simulink model "airgk"  (Simulink 8.7)
settings: Solver=ode45  StartTime=0  StopTime=250  RelTol=1e-3
undefined symbols (not defined in the file or in its folder): GM1, x0, xfix
undefined symbols (not defined in the file): AM, GM2
libraries: airlib x1
(part 2 of 2)

== system airgk/Subsystem/eqm/xdotcorr ==
  xdot uncorrected : Inport
  yhlp : Inport  Port=2
  yatm : Inport  Port=3
  0 : Subsystem
      mask Display: disp('XDOTCORR (General)\nM.O. Rauw, October 1997')
  Demux : Demux  Outputs=12
  Mux1 : Mux  Inputs=12
  Mux2 : Mux  Inputs=[11 1 5]
  beta dot correction : Fcn  Expr=u[12] / (1 - (u[3]*u[13]*b*S*CYbdot)/(4*m))
  xdot corrected : Outport
  wires:
  beta dot correction/1 -> Mux1/3
  yatm/1 -> Mux2/3
  Demux/1 -> Mux1/1
  Demux/2 -> Mux1/2
  Demux/4 -> Mux1/4
  Demux/5 -> Mux1/5
  Demux/6 -> Mux1/6
  Demux/7 -> Mux1/7
  Demux/8 -> Mux1/8
  Demux/9 -> Mux1/9
  Demux/10 -> Mux1/10
  Demux/11 -> Mux1/11
  Demux/12 -> Mux1/12
  Demux/3 -> Mux2/2
  xdot uncorrected/1 -> Demux/1
  Mux1/1 -> xdot corrected/1
  Mux2/1 -> beta dot correction/1
  yhlp/1 -> Mux2/1

== system airgk/Subsystem/fms/0 ==

== system airgk/Subsystem/fw/0 ==

== system airgk/Subsystem/gr/0 ==

== system airgk/Subsystem/hlp/0 ==

== system airgk/Subsystem/out/0 ==

== system airgk/Subsystem/out/accel ==
  Ftot : Inport
  Fgrav : Inport  Port=2
  0 : Subsystem
      mask Display: disp('ACCEL\nM.O. Rauw, October 1997')
  Ax : Fcn  Expr=(u[1]-u[4])/(m*9.80665)
  Ay : Fcn  Expr=(u[2]-u[5])/(m*9.80665)
  Az : Fcn  Expr=(u[3]-u[6])/(m*9.80665)
  Mux : Mux  Inputs=6
  Mux1 : Mux  Inputs=[3 3]
  axk : Fcn  Expr=u[1]/(m*9.80665)
  ayk : Fcn  Expr=u[2]/(m*9.80665)
  azk : Fcn  Expr=u[3]/(m*9.80665)
  yacc : Outport
  wires:
  Ftot/1 -> Mux1/1
  Fgrav/1 -> Mux1/2
  Mux/1 -> yacc/1
  azk/1 -> Mux/6
  Az/1 -> Mux/3
  Ay/1 -> Mux/2
  Ax/1 -> Mux/1
  Mux1/1 -> Az/1, Ax/1, Ay/1, axk/1, azk/1, ayk/1
  axk/1 -> Mux/4
  ayk/1 -> Mux/5

== system airgk/Subsystem/out/fp ==
  x : Inport
  xdot : Inport  Port=2
  0 : Subsystem
      mask Display: disp('FLPATH\nM.O. Rauw, October 1997')
  Mux : Mux  Inputs=[12 12]
  Mux1 : Mux
  Phi : Fcn  Expr=u[9]*cos(u[8]-alpha0)
  chi : Fcn  Expr=u[3]+u[7]
  fpa : Fcn  Expr=u[13]/9.80665
  gamma : Fcn  Expr=asin(u[24]/u[1])
  yfp : Outport
  wires:
  gamma/1 -> Mux1/1
  Mux/1 -> chi/1, Phi/1, fpa/1, gamma/1
  fpa/1 -> Mux1/2
  chi/1 -> Mux1/3
  Phi/1 -> Mux1/4
  Mux1/1 -> yfp/1
  x/1 -> Mux/1
  xdot/1 -> Mux/2

== system airgk/Subsystem/out/uvwdot ==
  note: `
  note: cos(alpha)
  note: sin(alpha)
  note: cos(beta)
  note: sin(beta)
  note: V
  x : Inport
  xdot : Inport  Port=2
  yhlp : Inport  Port=3
  0 : Subsystem
      mask Display: disp('UVWDOT\nM.O. Rauw, October 1997')
  DeMux : Demux  Outputs=[1 1 1 1 7]
  Demux : Demux  Outputs=[1 11]
  Mux : Mux  Inputs=[1 1 1 1 1 12]
  Mux1 : Mux  Inputs=3
  Terminator : Terminator
  Terminator1 : Terminator
  u dot : Fcn  Expr=u[6]*u[1]*u[3] - u[5]*(u[7]*u[2]*u[3] + u[8]*u[1]*u[4])
  v dot : Fcn  Expr=u[6]*u[4] + u[5]*u[3]*u[8]
  wdot : Fcn  Expr=u[6]*u[2]*u[3] + u[5]*(u[7]*u[1]*u[3] - u[8]*u[2]*u[4])
  yuvw =  [udot; vdot; wdot] : Outport
  wires:
  Demux/2 -> Terminator1/1
  DeMux/5 -> Terminator/1
  wdot/1 -> Mux1/3
  v dot/1 -> Mux1/2
  u dot/1 -> Mux1/1
  xdot/1 -> Mux/6
  Mux/1 -> v dot/1, wdot/1, u dot/1
  DeMux/1 -> Mux/1
  DeMux/2 -> Mux/2
  x/1 -> Demux/1
  Mux1/1 -> yuvw =  [udot; vdot; wdot]/1
  yhlp/1 -> DeMux/1
  DeMux/3 -> Mux/3
  DeMux/4 -> Mux/4
  Demux/1 -> Mux/5

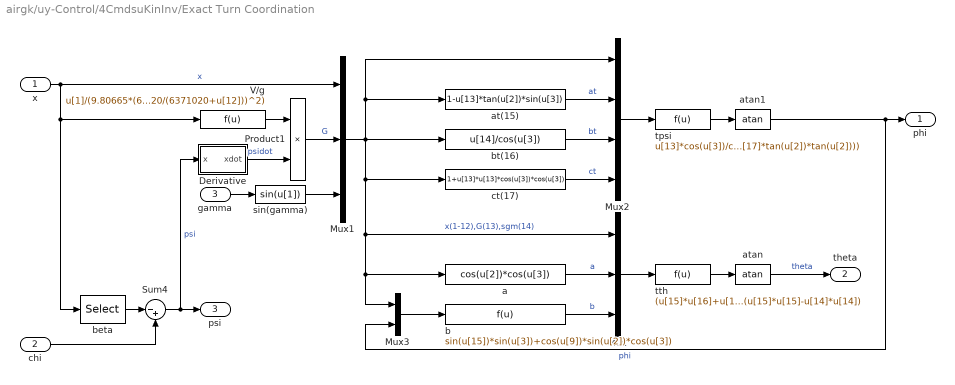
== system airgk/uy-Control/4CmdsuKinInv/Exact Turn Coordination ==
  x : Inport
  chi : Inport  Port=2
  gamma : Inport  Port=3
  Derivative : Subsystem  mask(Time Derivative){T=T, x0=Psi0}
      mask prompts: T "Sampling Time"; x0 "Initial Condition"
      mask help:
      | First order approximation of the time derivative of the input signal,
      |   the original one is buggy.
  Mux : Mux  Inputs=[14 1 1]
  Mux1 : Mux  Inputs=[12 1 1]
  Mux2 : Mux  Inputs=[14 1 1 1]
  Mux3 : Mux  Inputs=[14 1]
  Product1 : Product  Inputs=**  SaturateOnIntegerOverflow=on  RndMeth=Zero  InputSameDT=on  OutDataTypeStr=Inherit: Same as first input
  Sum4 : Sum  Inputs=|-+  SaturateOnIntegerOverflow=on  InputSameDT=on  OutDataTypeStr=Inherit: Same as first input
  V/g : Fcn  Expr=u[1]/(9.80665*(6371020/(6371020+u[12]))^2)
  a : Fcn  Expr=cos(u[2])*cos(u[3])
  at(15) : Fcn  Expr=1-u[13]*tan(u[2])*sin(u[3])
  atan : Trigonometry  Operator=atan
  atan1 : Trigonometry  Operator=atan
  b : Fcn  Expr=sin(u[15])*sin(u[3])+cos(u[9])*sin(u[2])*cos(u[3])
  beta : Selector  InputPortWidth=12  IndexOptions=Index vector (dialog)  Indices=3  OutputSizes=1
  bt(16) : Fcn  Expr=u[14]/cos(u[3])
  ct(17) : Fcn  Expr=1+u[13]*u[13]*cos(u[3])*cos(u[3])
  sin(gamma) : Fcn
  tpsi : Fcn  Expr=u[13]*cos(u[3])/cos(u[2])*(u[15]-u[16]*u[16]+u[16]*tan(u[2])*sqrt(abs(u[17]*(1-u[16]*u[16])+u[13]*u[13]*sin(u[3])*sin(u[3]))))/(u[15]*u[15]-u[16]*u[16]*(1+u[17]*tan(u[2])*tan(u[2])))
  tth : Fcn  Expr=(u[15]*u[16]+u[14]*sqrt(abs(u[15]*u[15]-u[14]*u[14]+u[16]*u[16])))/(u[15]*u[15]-u[14]*u[14])
  phi : Outport
  theta : Outport  Port=2
  psi : Outport  Port=3
  wires:
  Sum4/1 -> Derivative/1(x), psi/1  "psi"
  beta/1 -> Sum4/1
  chi/1 -> Sum4/2
  Derivative/1(xdot) -> Product1/2  "psidot"
  V/g/1 -> Product1/1
  gamma/1 -> sin(gamma)/1
  sin(gamma)/1 -> Mux1/3
  Product1/1 -> Mux1/2  "G"
  Mux1/1 -> bt(16)/1, at(15)/1, Mux2/1, ct(17)/1, Mux/1, a/1, Mux3/1  "x(1-12),G(13),sgm(14)"
  Mux2/1 -> tpsi/1
  tth/1 -> atan/1
  Mux/1 -> tth/1
  Mux3/1 -> b/1
  a/1 -> Mux/2  "a"
  b/1 -> Mux/3  "b"
  atan1/1 -> Mux3/2, phi/1  "phi"
  tpsi/1 -> atan1/1
  at(15)/1 -> Mux2/2  "at"
  bt(16)/1 -> Mux2/3  "bt"
  ct(17)/1 -> Mux2/4  "ct"
  atan/1 -> theta/1  "theta"
  x/1 -> beta/1, V/g/1, Mux1/1  "x"

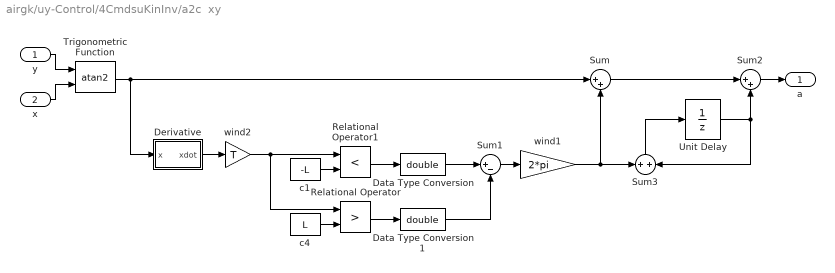
== system airgk/uy-Control/4CmdsuKinInv/a2c  xy ==
  y : Inport
  x : Inport  Port=2
  Data Type Conversion : DataTypeConversion  OutDataTypeStr=double  SaturateOnIntegerOverflow=on  RndMeth=Zero
  Data Type Conversion1 : DataTypeConversion  OutDataTypeStr=double  SaturateOnIntegerOverflow=on  RndMeth=Zero
  Derivative : Subsystem  mask(Time Derivative){T=T}
      mask prompts: T "Sampling Time"
      mask help:
      | First order approximation of the time derivative of the input signal,
      |   the original one is buggy.
  Relational Operator : RelationalOperator  Operator=>  InputSameDT=on
  Relational Operator1 : RelationalOperator  Operator=<  InputSameDT=on
  Sum : Sum  Inputs=|++  SaturateOnIntegerOverflow=on  InputSameDT=on  OutDataTypeStr=Inherit: Same as first input
  Sum1 : Sum  Inputs=|+-  SaturateOnIntegerOverflow=on  InputSameDT=on  OutDataTypeStr=Inherit: Same as first input
  Sum2 : Sum  Inputs=|++  SaturateOnIntegerOverflow=on  InputSameDT=on  OutDataTypeStr=Inherit: Same as first input
  Sum3 : Sum  SaturateOnIntegerOverflow=on  InputSameDT=on  OutDataTypeStr=Inherit: Same as first input
  Trigonometric Function : Trigonometry  Operator=atan2
  Unit Delay : UnitDelay  SampleTime=T
  c1 : Constant  Value=-L
  c4 : Constant  Value=L
  wind1 : Gain  Gain=2*pi  SaturateOnIntegerOverflow=on  OutDataTypeStr=Inherit: Same as input  ParamDataTypeStr=Inherit: Same as input
  wind2 : Gain  Gain=T  SaturateOnIntegerOverflow=on  OutDataTypeStr=Inherit: Same as input  ParamDataTypeStr=Inherit: Same as input
  a : Outport
  wires:
  Trigonometric Function/1 -> Sum/1, Derivative/1(x)
  Derivative/1(xdot) -> wind2/1
  wind2/1 -> Relational Operator/1, Relational Operator1/1
  c4/1 -> Relational Operator/2
  c1/1 -> Relational Operator1/2
  Relational Operator1/1 -> Data Type Conversion/1
  Relational Operator/1 -> Data Type Conversion1/1
  Data Type Conversion/1 -> Sum1/1
  Data Type Conversion1/1 -> Sum1/2
  Sum1/1 -> wind1/1
  wind1/1 -> Sum/2, Sum3/1
  Sum/1 -> Sum2/1
  Unit Delay/1 -> Sum2/2, Sum3/2
  Sum3/1 -> Unit Delay/1
  y/1 -> Trigonometric Function/1
  Sum2/1 -> a/1
  x/1 -> Trigonometric Function/2

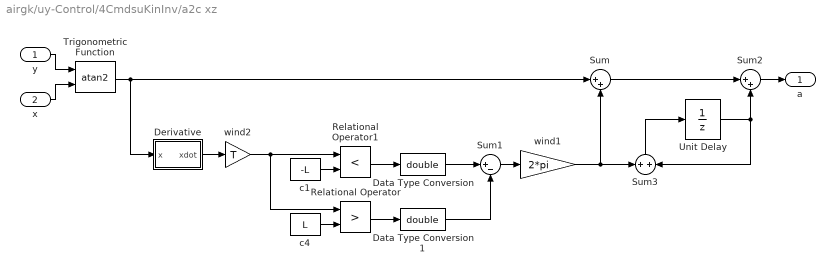
== system airgk/uy-Control/4CmdsuKinInv/a2c xz ==
  y : Inport
  x : Inport  Port=2
  Data Type Conversion : DataTypeConversion  OutDataTypeStr=double  SaturateOnIntegerOverflow=on  RndMeth=Zero
  Data Type Conversion1 : DataTypeConversion  OutDataTypeStr=double  SaturateOnIntegerOverflow=on  RndMeth=Zero
  Derivative : Subsystem  mask(Time Derivative){T=T}
      mask prompts: T "Sampling Time"
      mask help:
      | First order approximation of the time derivative of the input signal,
      |   the original one is buggy.
  Relational Operator : RelationalOperator  Operator=>  InputSameDT=on
  Relational Operator1 : RelationalOperator  Operator=<  InputSameDT=on
  Sum : Sum  Inputs=|++  SaturateOnIntegerOverflow=on  InputSameDT=on  OutDataTypeStr=Inherit: Same as first input
  Sum1 : Sum  Inputs=|+-  SaturateOnIntegerOverflow=on  InputSameDT=on  OutDataTypeStr=Inherit: Same as first input
  Sum2 : Sum  Inputs=|++  SaturateOnIntegerOverflow=on  InputSameDT=on  OutDataTypeStr=Inherit: Same as first input
  Sum3 : Sum  SaturateOnIntegerOverflow=on  InputSameDT=on  OutDataTypeStr=Inherit: Same as first input
  Trigonometric Function : Trigonometry  Operator=atan2
  Unit Delay : UnitDelay  SampleTime=T
  c1 : Constant  Value=-L
  c4 : Constant  Value=L
  wind1 : Gain  Gain=2*pi  SaturateOnIntegerOverflow=on  OutDataTypeStr=Inherit: Same as input  ParamDataTypeStr=Inherit: Same as input
  wind2 : Gain  Gain=T  SaturateOnIntegerOverflow=on  OutDataTypeStr=Inherit: Same as input  ParamDataTypeStr=Inherit: Same as input
  a : Outport
  wires:
  x/1 -> Trigonometric Function/2
  Sum2/1 -> a/1
  y/1 -> Trigonometric Function/1
  Sum3/1 -> Unit Delay/1
  Unit Delay/1 -> Sum3/2, Sum2/2
  Sum/1 -> Sum2/1
  wind1/1 -> Sum3/1, Sum/2
  Sum1/1 -> wind1/1
  Data Type Conversion1/1 -> Sum1/2
  Data Type Conversion/1 -> Sum1/1
  Relational Operator/1 -> Data Type Conversion1/1
  Relational Operator1/1 -> Data Type Conversion/1
  c1/1 -> Relational Operator1/2
  c4/1 -> Relational Operator/2
  wind2/1 -> Relational Operator1/1, Relational Operator/1
  Derivative/1(xdot) -> wind2/1
  Trigonometric Function/1 -> Derivative/1(x), Sum/1

== system airgk/uy-Control/Vcmd Generator/IIR1 ==
  In : Inport
  Discrete State-Space : DiscreteStateSpace  A=A  B=B  C=C  D=D  X0=x0  SampleTime=T
  Out : Outport
  wires:
  In/1 -> Discrete State-Space/1
  Discrete State-Space/1 -> Out/1

== system airgk/uy-Control/Vcmd Generator/IIR2 ==
  In : Inport
  Discrete State-Space : DiscreteStateSpace  A=A  B=B  C=C  D=D  X0=x0  SampleTime=T
  Out : Outport
  wires:
  In/1 -> Discrete State-Space/1
  Discrete State-Space/1 -> Out/1

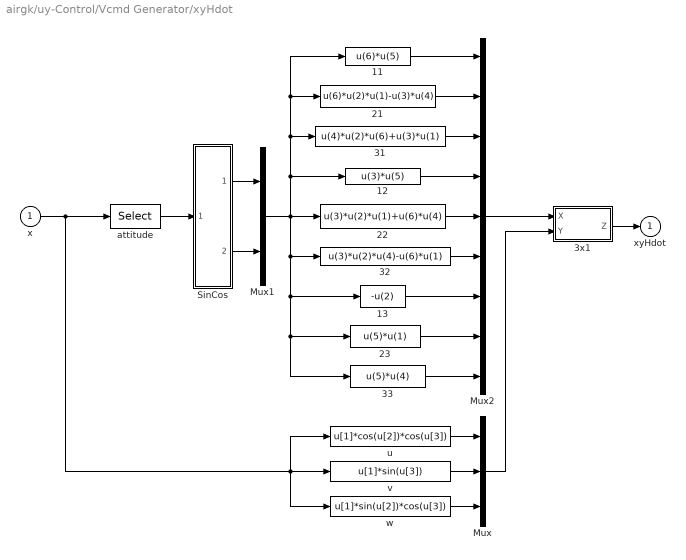
== system airgk/uy-Control/Vcmd Generator/xyHdot ==
  x : Inport
  11 : Fcn  Expr=u(6)*u(5)
  12 : Fcn  Expr=u(3)*u(5)
  13 : Fcn  Expr=-u(2)
  21 : Fcn  Expr=u(6)*u(2)*u(1)-u(3)*u(4)
  22 : Fcn  Expr=u(3)*u(2)*u(1)+u(6)*u(4)
  23 : Fcn  Expr=u(5)*u(1)
  31 : Fcn  Expr=u(4)*u(2)*u(6)+u(3)*u(1)
  32 : Fcn  Expr=u(3)*u(2)*u(4)-u(6)*u(1)
  33 : Fcn  Expr=u(5)*u(4)
  3x1 : Subsystem  mask(3x3 Matrix Multiplication){}
      mask help:
      | Input 1   : elements of matrix X (3 by 3)
      |   Input 2   : elements of matrix Y (3 by 3)
      |   Output   : elements of matrix X*Y (3 by 3)
      mask Help:
      | <p>
      | Elements of input and output matrices are taken columnwise.
      | </p>
      mask Display: disp('Z=X*Y')
  Mux : Mux  Inputs=3
  Mux1 : Mux  Inputs=2
  Mux2 : Mux  Inputs=9
  SinCos : Subsystem  mask(SinCos){}
      mask help: Compute the sine and cosine of input, u. u is in radians.
      mask Help: web(asbhelp);
      mask Display:
      | port_label('output',1,'sin(u)','texmode','on');
      | port_label('output',2,'cos(u)','texmode','on');
  attitude : Selector  InputPortWidth=12  IndexOptions=Index vector (dialog)  Indices=[9 8 7]  OutputSizes=1
  u : Fcn  Expr=u[1]*cos(u[2])*cos(u[3])
  v : Fcn  Expr=u[1]*sin(u[3])
  w : Fcn  Expr=u[1]*sin(u[2])*cos(u[3])
  xyHdot : Outport
  wires:
  x/1 -> attitude/1, v/1, w/1, u/1
  33/1 -> Mux2/9
  23/1 -> Mux2/8
  13/1 -> Mux2/7
  32/1 -> Mux2/6
  22/1 -> Mux2/5
  12/1 -> Mux2/4
  31/1 -> Mux2/3
  21/1 -> Mux2/2
  11/1 -> Mux2/1
  SinCos/1(sin(theta)) -> Mux1/1
  SinCos/2(cos(theta)) -> Mux1/2
  Mux1/1 -> 22/1, 11/1, 21/1, 31/1, 12/1, 32/1, 13/1, 23/1, 33/1
  attitude/1 -> SinCos/1(theta)
  w/1 -> Mux/3
  u/1 -> Mux/1
  v/1 -> Mux/2
  Mux/1 -> 3x1/2(Y)
  Mux2/1 -> 3x1/1(X)
  3x1/1(Z) -> xyHdot/1

== system airgk/uy-Control/uDynInv/ u term ==
  x : Inport
  udd : Inport  Port=2
  Mux1 : Mux  Inputs=[12 3 1]
  Term 1 with T=0 : Fcn  Expr=m*u[12+4]+m*(9.80665*(6371020/(6371020+u[12]))^2)*sin(u[8])+m*(u[5]*u[12+3]-u[6]*u[12+2])
  uvw : Subsystem  mask(uvw){}
      mask help:
      | Calculation of body-axes velocities
      | u, v, and w
      mask Help: eval('fdchelp uvw')
      mask Display: disp('Body-axes\nvelocities')
  mix : Outport
  wires:
  x/1 -> Mux1/1, uvw/1(x)
  Mux1/1 -> Term 1 with T=0/1
  Term 1 with T=0/1 -> mix/1
  uvw/1(ybvel) -> Mux1/2
  udd/1 -> Mux1/3

== system airgk/uy-Control/uDynInv/AM_CF ==
  In1 : Inport
  Matrix Gain : StateSpace  A=[]  B=[]  C=[]  D=M  X0=0
  Out1 : Outport
  wires:
  In1/1 -> Matrix Gain/1
  Matrix Gain/1 -> Out1/1

== system airgk/uy-Control/uDynInv/AM_SF ==
  In1 : Inport
  Matrix Gain : StateSpace  A=[]  B=[]  C=[]  D=M  X0=0
  Out1 : Outport
  wires:
  In1/1 -> Matrix Gain/1
  Matrix Gain/1 -> Out1/1

== system airgk/uy-Control/uDynInv/AM_SM ==
  In1 : Inport
  Matrix Gain : StateSpace  A=[]  B=[]  C=[]  D=M  X0=0
  Out1 : Outport
  wires:
  Matrix Gain/1 -> Out1/1
  In1/1 -> Matrix Gain/1

== system airgk/uy-Control/uDynInv/Inertia Products ==
  w : Inport
  wd : Inport  Port=2
  3x1mult : Subsystem  mask(3x1 Matrix Multiplication){}
      mask help:
      | Input 1   : elements of matrix X (3 by 3)
      |   Input 2   : elements of matrix Y (3 by 1)
      |   Output   : elements of matrix X*Y (3 by 1)
      mask Help:
      | <p>
      | Elements of input and output matrices are taken columnwise.
      | </p>
      mask Display: disp('Z=X*Y')
  3x1mult1 : Subsystem  mask(3x1 Matrix Multiplication){}
      mask help:
      | Input 1   : elements of matrix X (3 by 3)
      |   Input 2   : elements of matrix Y (3 by 1)
      |   Output   : elements of matrix X*Y (3 by 1)
      mask Help:
      | <p>
      | Elements of input and output matrices are taken columnwise.
      | </p>
      mask Display: disp('Z=X*Y')
  3x1mult2 : Subsystem  mask(3x1 Matrix Multiplication){}
      mask help:
      | Input 1   : elements of matrix X (3 by 3)
      |   Input 2   : elements of matrix Y (3 by 1)
      |   Output   : elements of matrix X*Y (3 by 1)
      mask Help:
      | <p>
      | Elements of input and output matrices are taken columnwise.
      | </p>
      mask Display: disp('Z=X*Y')
  Inertia Matrix : Constant  Value=[GM1(4) -GM1(7) -GM1(8) -GM1(7) GM1(5) -GM1(9) -GM1(8) -GM1(9) GM1(6)]
  Sum : Sum  Inputs=|++  SaturateOnIntegerOverflow=on  InputSameDT=on  OutDataTypeStr=Inherit: Same as first input
  w2W : Subsystem
      mask Display: disp('S')
  W*J*w+J*wt : Outport
  wires:
  w2W/1(Out1) -> 3x1mult2/1(X)
  3x1mult1/1(Z) -> 3x1mult2/2(Y)
  w/1 -> 3x1mult1/2(Y), w2W/1(In1)
  3x1mult/1(Z) -> Sum/1
  3x1mult2/1(Z) -> Sum/2
  Sum/1 -> W*J*w+J*wt/1
  wd/1 -> 3x1mult/2(Y)
  Inertia Matrix/1 -> 3x1mult/1(X), 3x1mult1/1(X)

== system airgk/uy-Control/uDynInv/Inv Rot ==
  w : Inport
  ftp : Inport  Port=2
  add : Inport  Port=3
  M : Subsystem  mask(Simulink Matrix Library Block){}
      mask help:
      | Roll, Pitch and Yaw derivatives to Omega :
      |   Input 1 : Roll, Pitch and Yaw angles (phi,theta,psi)
      |   Input 2 : Roll, Pitch and Yaw derivatives
      |   Output : Omega (p,q,r)
      mask Help:
      | <p>
      | Roll, Pitch and Yaw angles express the orientation
      | of the Body frame with respect to the Earth frame.
      | </p>
      | <p>
      | To use this block you should have the smxl library in your path.
      | </p>
  Sum1 : Sum  Inputs=+++  SaturateOnIntegerOverflow=on  InputSameDT=on  OutDataTypeStr=Inherit: Same as first input
  dM/df : Subsystem
  dM/dt : Subsystem
  pqr2ftpdot : Subsystem  mask(Simulink Matrix Library Block){}
      mask help:
      | Omega to Roll, Pitch and Yaw derivatives :
      |   Input 1 : Roll, Pitch and Yaw angles (phi,theta,psi)
      |   Input 2 : Omega (p,q,r)
      |   Output : Roll, Pitch and Yaw derivatives
      mask Help:
      | <p>
      | Roll, Pitch and Yaw angles express the orientation
      | of the Body frame with respect to the Earth frame.
      | </p>
      | <p>
      | To use this block you should have the smxl library in your path.
      | </p>
  wd : Outport
  wires:
  add/1 -> M/2(ftpdot)
  ftp/1 -> pqr2ftpdot/1(ftp), M/1(ftp), dM/df/1(ftp), dM/dt/1(ftp)
  w/1 -> pqr2ftpdot/2(pqr)
  pqr2ftpdot/1(ftpdot) -> dM/dt/2(ftpd), dM/df/2(ftpd)
  M/1(pqr) -> Sum1/3
  dM/dt/1(Tt) -> Sum1/1
  dM/df/1(Tf) -> Sum1/2
  Sum1/1 -> wd/1

== system airgk/uy-Control/uDynInv/ad1 ==
  x : Inport
  yatm : Inport  Port=2
  0 : Subsystem
      settings: OpenFcn=fdchelp airdata1
      mask Display: disp('AIRDATA1\nM.O. Rauw, October 1997')
  M : Fcn  Expr=u[2]/u[1]
  Mux : Mux  Inputs=[1 12]
  Mux1 : Mux  Inputs=[12 5]
  Mux2 : Mux  Inputs=3
  a : Fcn  Expr=sqrt(401.8743*u[3])
  qdyn : Fcn  Expr=0.5*u[13]*u[1]^2
  yad1 : Outport
  wires:
  yatm/1 -> Mux1/2, a/1
  x/1 -> Mux1/1, Mux/2
  Mux/1 -> M/1
  Mux1/1 -> qdyn/1
  M/1 -> Mux2/2
  a/1 -> Mux2/1, Mux/1
  qdyn/1 -> Mux2/3
  Mux2/1 -> yad1/1

== system airgk/uy-Control/uDynInv/atm ==
  x : Inport
  0 : Subsystem
      settings: OpenFcn=fdchelp atmosph
      mask Display: disp('ATMOSPH\nM.O. Rauw, October 1997')
  Mux : Mux  Inputs=2
  Mux1 : Mux  Inputs=[2 1]
  Mux2 : Mux  Inputs=5
  T : Fcn  Expr=288.15 - 0.0065*u[12]
  g : Fcn  Expr=9.80665*(6371020/(6371020+u[12]))^2
  mu : Fcn  Expr=(1.458*10^(-6)*u[2]^1.5)/(u[2]+110.4)
  ps : Fcn  Expr=101325*(u[2]/288.15)^(u[1]/1.86584)
  rho : Fcn  Expr=u[3]/(287.053*u[2])
  yatm : Outport
  wires:
  mu/1 -> Mux2/4
  Mux2/1 -> yatm/1
  Mux1/1 -> rho/1
  rho/1 -> Mux2/1
  g/1 -> Mux2/5, Mux/1
  T/1 -> Mux2/3, Mux/2
  ps/1 -> Mux2/2, Mux1/2
  Mux/1 -> ps/1, mu/1, Mux1/1
  x/1 -> g/1, T/1

== system airgk/uy-Control/uDynInv/dl ==
  x : Inport
  0 : Subsystem
      settings: OpenFcn=fdchelp dimless
      mask Display: disp('DIMLESS\nM.O. Rauw, October 1997')
  Mux : Mux  Inputs=3
  pb/2V : Fcn  Expr=0.5 * u[4] * b / u[1]
  qc/2V : Fcn  Expr=0.5* u[5] * cbar / u[1]
  rb/2V : Fcn  Expr=0.5 * u[6] * b / u[1]
  ydl : Outport
  wires:
  pb/2V/1 -> Mux/1
  qc/2V/1 -> Mux/2
  rb/2V/1 -> Mux/3
  Mux/1 -> ydl/1
  x/1 -> qc/2V/1, rb/2V/1, pb/2V/1

== system airgk/uy-Control/uDynInv/inv AM_CM ==
  In1 : Inport
  Matrix Gain : StateSpace  A=[]  B=[]  C=[]  D=M  X0=0
  Out1 : Outport
  wires:
  In1/1 -> Matrix Gain/1
  Matrix Gain/1 -> Out1/1

== system airgk/Subsystem/ad/ad1/0 ==

== system airgk/Subsystem/ad/atm/0 ==

== system airgk/Subsystem/ae/aero/0 ==

== system airgk/Subsystem/ae/aero/AM  ==
  In1 : Inport
  Matrix Gain : StateSpace  A=[]  B=[]  C=[]  D=M  X0=0
  Out1 : Outport
  wires:
  In1/1 -> Matrix Gain/1
  Matrix Gain/1 -> Out1/1

== system airgk/Subsystem/ae/aero/Stability 2 Body Axis ==
  alpha : Inport
  FsMb : Inport  Port=2
  Demux2 : Demux  Outputs=6
  Mux1 : Mux  Inputs=6
  Product{2..5} (4 alike) : Product  SaturateOnIntegerOverflow=on  RndMeth=Zero  InputSameDT=on  OutDataTypeStr=Inherit: Same as first input
  Sum3 : Sum  Inputs=-+  SaturateOnIntegerOverflow=on  InputSameDT=on  OutDataTypeStr=Inherit: Same as first input
  Sum4 : Sum  Inputs=--  SaturateOnIntegerOverflow=on  InputSameDT=on  OutDataTypeStr=Inherit: Same as first input
  cos alpha : Fcn  Expr=cos(u[1])
  sin alpha : Fcn
  FbMb : Outport
  wires:
  Demux2/6 -> Mux1/6
  Demux2/5 -> Mux1/5
  Demux2/2 -> Mux1/2
  Demux2/4 -> Mux1/4
  cos alpha/1 -> Product2/1, Product5/1
  Demux2/1 -> Product2/2, Product4/2
  Product2/1 -> Sum3/1
  Product3/1 -> Sum3/2
  Sum3/1 -> Mux1/1
  sin alpha/1 -> Product3/1, Product4/1
  Demux2/3 -> Product3/2, Product5/2
  Product4/1 -> Sum4/1
  Product5/1 -> Sum4/2
  Sum4/1 -> Mux1/3
  alpha/1 -> sin alpha/1, cos alpha/1
  Mux1/1 -> FbMb/1
  FsMb/1 -> Demux2/1

== system airgk/Subsystem/ae/dl/0 ==

== system airgk/Subsystem/ae/fmdims/0 ==

== system airgk/Subsystem/eqm/ODE/0 ==

== system airgk/Subsystem/eqm/ODE/Eulerdot ==
  note: ueul=[x;Ftot;Mtot;yhlp]
  note: yeul=[psi dot; theta dot; phi dot]
  ueul : Inport
  0 : Subsystem
      mask Display: disp('EULERDOT\nM.O. Rauw, October 1997')
  Mux1 : Mux  Inputs=[29 1]
  Mux2 : Mux  Inputs=3
  phi dot : Fcn  Expr=u[4] + u[30]*u[26]
  psi dot : Fcn  Expr=(u[5]*u[28] + u[6]*u[29])/u[27]
  theta dot : Fcn  Expr=u[5]*u[29] - u[6]*u[28]
  yeul : Outport
  wires:
  ueul/1 -> theta dot/1, Mux1/1, psi dot/1
  psi dot/1 -> Mux2/1, Mux1/2
  theta dot/1 -> Mux2/2
  Mux2/1 -> yeul/1
  phi dot/1 -> Mux2/3
  Mux1/1 -> phi dot/1

== system airgk/Subsystem/eqm/ODE/Vabdot ==
  note: yVab=[V dot;alpha dot;beta dot]
  note: uVab=[x;Ftot;Mtot;yhlp]
  uVab : Inport
  0 : Subsystem
      mask Display: disp('VABDOT\nM.O. Rauw, October 1997')
  Mux2 : Mux  Inputs=3
  V dot : Fcn  Expr=(u[13]*u[19]*u[21]+u[14]*u[22]+u[15]*u[20]*u[21])/m
  alpha dot : Fcn  Expr=(-u[13]*u[20]+u[15]*u[19])/(m*u[1]*u[21]) - u[23]*(u[4]*u[19]+u[6]*u[20]) + u[5]
  beta dot : Fcn  Expr=(-u[13]*u[19]*u[22]+u[14]*u[21]-u[15]*u[20]*u[22])/(m*u[1]) + u[4]*u[20] - u[6]*u[19]
  yVab : Outport
  wires:
  beta dot/1 -> Mux2/3
  V dot/1 -> Mux2/1
  alpha dot/1 -> Mux2/2
  uVab/1 -> alpha dot/1, beta dot/1, V dot/1
  Mux2/1 -> yVab/1

== system airgk/Subsystem/eqm/ODE/pqrdot ==
  note: ytmp = [L; M; N; p^2; pq; pr; q^2; qr; r^2]
  note: upqr=[x;Ftot;Mtot;yhlp]
  note: ypqr=[p dot;q dot;r dot]
  note: ytmp
  note: Here: ypqr = GM2*ytmp
  note: [L M N]'
  note: [p q r]'
  upqr : Inport
  0 : Subsystem
      mask Display: disp('PQRDOT\nM.O. Rauw, October 1997')
  Demux : Demux  Outputs=[3 3 9 3 11]
  Fcn : Fcn  Expr=u[1]^2
  Fcn1 : Fcn  Expr=u[1]*u[2]
  Fcn2 : Fcn  Expr=u[1]*u[3]
  Fcn3 : Fcn  Expr=u[2]^2
  Fcn4 : Fcn  Expr=u[2]*u[3]
  Fcn5 : Fcn  Expr=u[3]^2
  "GM2 " : Subsystem  mask(State Space){M=GM2}
      mask prompts: M "Matrix"
      mask Display: disp('Matrix\nGain')
  Mux : Mux  Inputs=[3 1 1 1 1 1 1]
  Terminator1 : Terminator
  Terminator2 : Terminator
  Terminator3 : Terminator
  ypqr : Outport
  wires:
  Mux/1 -> "GM2 "/1(In1)
  "GM2 "/1(Out1) -> ypqr/1
  Fcn5/1 -> Mux/7
  Fcn4/1 -> Mux/6
  Fcn3/1 -> Mux/5
  Fcn2/1 -> Mux/4
  Fcn1/1 -> Mux/3
  Fcn/1 -> Mux/2
  Demux/4 -> Mux/1
  Demux/2 -> Fcn3/1, Fcn5/1, Fcn4/1, Fcn2/1, Fcn/1, Fcn1/1
  Demux/3 -> Terminator1/1
  Demux/5 -> Terminator2/1
  Demux/1 -> Terminator3/1
  upqr/1 -> Demux/1

== system airgk/Subsystem/eqm/ODE/xyHdot ==
  note: uxyH=[x;Ftot;Mtot;yhlp]
  note: yxyH=[xe dot; ye dot; H dot]
  ybvel* : Inport
  uxYH : Inport  Port=2
  0 : Subsystem
      mask Display: disp('XYHDOT\nM.O. Rauw, October 1997')
  H dot : Fcn  Expr=u[30]*u[26] - (u[31]*u[28]+u[32]*u[29])*u[27]
  Mux2 : Mux  Inputs=[29 3]
  Mux3 : Mux  Inputs=2
  Mux4 : Mux  Inputs=[29 2]
  Mux5 : Mux  Inputs=3
  tmp1 : Fcn  Expr=u[30]*u[27] + (u[31]*u[28]+u[32]*u[29])*u[26]
  tmp2 : Fcn  Expr=u[31]*u[29] - u[32]*u[28]
  xe dot : Fcn  Expr=u[30]*u[25] - u[31]*u[24]
  ye dot : Fcn  Expr=u[30]*u[24] + u[31]*u[25]
  yxyH : Outport
  wires:
  uxYH/1 -> Mux2/1, Mux4/1
  ybvel*/1 -> Mux2/2
  Mux3/1 -> Mux4/2
  Mux2/1 -> tmp1/1, tmp2/1, H dot/1
  Mux4/1 -> xe dot/1, ye dot/1
  Mux5/1 -> yxyH/1
  ye dot/1 -> Mux5/2
  tmp2/1 -> Mux3/2
  xe dot/1 -> Mux5/1
  H dot/1 -> Mux5/3
  tmp1/1 -> Mux3/1

== system airgk/Subsystem/eqm/uvw/0 ==

== system airgk/Subsystem/eqm/xdotcorr/0 ==

== system airgk/Subsystem/out/accel/0 ==

== system airgk/Subsystem/out/fp/0 ==

== system airgk/Subsystem/out/uvwdot/0 ==

== system airgk/uy-Control/4CmdsuKinInv/Exact Turn Coordination/Derivative ==
  x : Inport
  Product2 : Product  Inputs=/*  SaturateOnIntegerOverflow=on  RndMeth=Zero  InputSameDT=on  OutDataTypeStr=Inherit: Same as first input
  Sum4 : Sum  Inputs=|+-  SaturateOnIntegerOverflow=on  InputSameDT=on  OutDataTypeStr=Inherit: Same as first input
  Unit Delay1 : UnitDelay  InitialCondition=x0  SampleTime=T
  Zero-Order Hold1 : ZeroOrderHold  SampleTime=T
  m : Constant  Value=T
  xdot : Outport
  wires:
  Sum4/1 -> Product2/2
  Unit Delay1/1 -> Sum4/2
  Zero-Order Hold1/1 -> Sum4/1, Unit Delay1/1
  m/1 -> Product2/1
  Product2/1 -> xdot/1
  x/1 -> Zero-Order Hold1/1

== system airgk/uy-Control/4CmdsuKinInv/a2c  xy/Derivative ==
  x : Inport
  Product2 : Product  Inputs=/*  SaturateOnIntegerOverflow=on  RndMeth=Zero  InputSameDT=on  OutDataTypeStr=Inherit: Same as first input
  Sum4 : Sum  Inputs=|+-  SaturateOnIntegerOverflow=on  InputSameDT=on  OutDataTypeStr=Inherit: Same as first input
  Unit Delay1 : UnitDelay  SampleTime=-1
  Zero-Order Hold1 : ZeroOrderHold  SampleTime=T
  m : Constant  Value=T
  xdot : Outport
  wires:
  x/1 -> Zero-Order Hold1/1
  Product2/1 -> xdot/1
  m/1 -> Product2/1
  Zero-Order Hold1/1 -> Unit Delay1/1, Sum4/1
  Unit Delay1/1 -> Sum4/2
  Sum4/1 -> Product2/2

== system airgk/uy-Control/4CmdsuKinInv/a2c xz/Derivative ==
  x : Inport
  Product2 : Product  Inputs=/*  SaturateOnIntegerOverflow=on  RndMeth=Zero  InputSameDT=on  OutDataTypeStr=Inherit: Same as first input
  Sum4 : Sum  Inputs=|+-  SaturateOnIntegerOverflow=on  InputSameDT=on  OutDataTypeStr=Inherit: Same as first input
  Unit Delay1 : UnitDelay  SampleTime=-1
  Zero-Order Hold1 : ZeroOrderHold  SampleTime=T
  m : Constant  Value=T
  xdot : Outport
  wires:
  Sum4/1 -> Product2/2
  Unit Delay1/1 -> Sum4/2
  Zero-Order Hold1/1 -> Sum4/1, Unit Delay1/1
  m/1 -> Product2/1
  Product2/1 -> xdot/1
  x/1 -> Zero-Order Hold1/1

== system airgk/uy-Control/Vcmd Generator/xyHdot/3x1 ==
  X : Inport
  Y : Inport  Port=2
  Dot Product1 : Subsystem  mask(Dot Product){}
      mask help:
      | Inner (dot) product.
      | y = sum(conj(u1).*u2). The operand u1 corresponds to the top (or left) input port.
      mask init:
      | t=(0:.1:2*pi)';
      | x=cos(t);
      | y=sin(t);
      | r=0.05;
      mask Help: Computes the inner (dot) product of the inputs: sum(u1.*u2).  The inputs are vectors of the same length. Output is a scalar.
      mask Display: patch([x*r+0.5],[y*r+0.5])
  Dot Product2 : Subsystem  mask(Dot Product){}
      mask help:
      | Inner (dot) product.
      | y = sum(conj(u1).*u2). The operand u1 corresponds to the top (or left) input port.
      mask init:
      | t=(0:.1:2*pi)';
      | x=cos(t);
      | y=sin(t);
      | r=0.05;
      mask Help: Computes the inner (dot) product of the inputs: sum(u1.*u2).  The inputs are vectors of the same length. Output is a scalar.
      mask Display: patch([x*r+0.5],[y*r+0.5])
  Dot Product9 : Subsystem  mask(Dot Product){}
      mask help:
      | Inner (dot) product.
      | y = sum(conj(u1).*u2). The operand u1 corresponds to the top (or left) input port.
      mask init:
      | t=(0:.1:2*pi)';
      | x=cos(t);
      | y=sin(t);
      | r=0.05;
      mask Help: Computes the inner (dot) product of the inputs: sum(u1.*u2).  The inputs are vectors of the same length. Output is a scalar.
      mask Display: patch([x*r+0.5],[y*r+0.5])
  Gain : Gain  Gain=-1  OutDataTypeStr=Inherit: Same as input  ParamDataTypeStr=Inherit: Same as input
  Mux : Mux  Inputs=3
  Selector : Selector  InputPortWidth=9  IndexOptions=Index vector (dialog)  Indices=[1:3]  OutputSizes=1
  Selector1 : Selector  InputPortWidth=9  IndexOptions=Index vector (dialog)  Indices=[4:6]  OutputSizes=1
  Selector2 : Selector  InputPortWidth=9  IndexOptions=Index vector (dialog)  Indices=[7:9]  OutputSizes=1
  Z : Outport
  wires:
  Mux/1 -> Z/1
  Selector2/1 -> Dot Product2/1(In1)
  Selector1/1 -> Dot Product1/1(In1)
  Y/1 -> Dot Product9/2(In2), Dot Product1/2(In2), Dot Product2/2(In2)
  Dot Product2/1(Out1) -> Gain/1
  Dot Product1/1(Out1) -> Mux/2
  Dot Product9/1(Out1) -> Mux/1
  Selector/1 -> Dot Product9/1(In1)
  X/1 -> Selector2/1, Selector1/1, Selector/1
  Gain/1 -> Mux/3

== system airgk/uy-Control/Vcmd Generator/xyHdot/SinCos ==
  theta : Inport
  cosine : Trigonometry  Operator=cos
  sine : Trigonometry
  sin(theta) : Outport
  cos(theta) : Outport  Port=2
  wires:
  cosine/1 -> cos(theta)/1
  sine/1 -> sin(theta)/1
  theta/1 -> cosine/1, sine/1

== system airgk/uy-Control/uDynInv/ u term/uvw ==
  x : Inport
  Mux : Mux  Inputs=3
  u : Fcn  Expr=u[1]*cos(u[2])*cos(u[3])
  v : Fcn  Expr=u[1]*sin(u[3])
  w : Fcn  Expr=u[1]*sin(u[2])*cos(u[3])
  ybvel : Outport
  wires:
  Mux/1 -> ybvel/1
  w/1 -> Mux/3
  v/1 -> Mux/2
  u/1 -> Mux/1
  x/1 -> v/1, w/1, u/1

== system airgk/uy-Control/uDynInv/Inertia Products/3x1mult ==
  X : Inport
  Y : Inport  Port=2
  Dot Product : DotProduct  OutDataTypeStr=Inherit: Inherit via internal rule
  Dot Product1 : DotProduct  OutDataTypeStr=Inherit: Inherit via internal rule
  Dot Product2 : DotProduct  OutDataTypeStr=Inherit: Inherit via internal rule
  Mux : Mux  Inputs=3
  Selector : Selector  InputPortWidth=9  IndexOptions=Index vector (dialog)  Indices=[0 3 6]+1  OutputSizes=1
  Selector1 : Selector  InputPortWidth=9  IndexOptions=Index vector (dialog)  Indices=[0 3 6]+2  OutputSizes=1
  Selector2 : Selector  InputPortWidth=9  IndexOptions=Index vector (dialog)  Indices=[0 3 6]+3  OutputSizes=1
  Z : Outport
  wires:
  Y/1 -> Dot Product/2, Dot Product1/2, Dot Product2/2
  Selector2/1 -> Dot Product2/1
  Selector1/1 -> Dot Product1/1
  Selector/1 -> Dot Product/1
  Mux/1 -> Z/1
  Dot Product2/1 -> Mux/3
  Dot Product1/1 -> Mux/2
  Dot Product/1 -> Mux/1
  X/1 -> Selector2/1, Selector1/1, Selector/1

== system airgk/uy-Control/uDynInv/Inertia Products/3x1mult1 ==
  X : Inport
  Y : Inport  Port=2
  Dot Product : DotProduct  OutDataTypeStr=Inherit: Inherit via internal rule
  Dot Product1 : DotProduct  OutDataTypeStr=Inherit: Inherit via internal rule
  Dot Product2 : DotProduct  OutDataTypeStr=Inherit: Inherit via internal rule
  Mux : Mux  Inputs=3
  Selector : Selector  InputPortWidth=9  IndexOptions=Index vector (dialog)  Indices=[0 3 6]+1  OutputSizes=1
  Selector1 : Selector  InputPortWidth=9  IndexOptions=Index vector (dialog)  Indices=[0 3 6]+2  OutputSizes=1
  Selector2 : Selector  InputPortWidth=9  IndexOptions=Index vector (dialog)  Indices=[0 3 6]+3  OutputSizes=1
  Z : Outport
  wires:
  Y/1 -> Dot Product/2, Dot Product1/2, Dot Product2/2
  Selector2/1 -> Dot Product2/1
  Selector1/1 -> Dot Product1/1
  Selector/1 -> Dot Product/1
  Mux/1 -> Z/1
  Dot Product2/1 -> Mux/3
  Dot Product1/1 -> Mux/2
  Dot Product/1 -> Mux/1
  X/1 -> Selector2/1, Selector1/1, Selector/1

== system airgk/uy-Control/uDynInv/Inertia Products/3x1mult2 ==
  X : Inport
  Y : Inport  Port=2
  Dot Product : DotProduct  OutDataTypeStr=Inherit: Inherit via internal rule
  Dot Product1 : DotProduct  OutDataTypeStr=Inherit: Inherit via internal rule
  Dot Product2 : DotProduct  OutDataTypeStr=Inherit: Inherit via internal rule
  Mux : Mux  Inputs=3
  Selector : Selector  InputPortWidth=9  IndexOptions=Index vector (dialog)  Indices=[0 3 6]+1  OutputSizes=1
  Selector1 : Selector  InputPortWidth=9  IndexOptions=Index vector (dialog)  Indices=[0 3 6]+2  OutputSizes=1
  Selector2 : Selector  InputPortWidth=9  IndexOptions=Index vector (dialog)  Indices=[0 3 6]+3  OutputSizes=1
  Z : Outport
  wires:
  Y/1 -> Dot Product/2, Dot Product1/2, Dot Product2/2
  Selector2/1 -> Dot Product2/1
  Selector1/1 -> Dot Product1/1
  Selector/1 -> Dot Product/1
  Mux/1 -> Z/1
  Dot Product2/1 -> Mux/3
  Dot Product1/1 -> Mux/2
  Dot Product/1 -> Mux/1
  X/1 -> Selector2/1, Selector1/1, Selector/1

== system airgk/uy-Control/uDynInv/Inertia Products/w2W ==
  In1 : Inport
  State Space : StateSpace  A=[]  B=[]  C=[]  D=[0 0 0;0 0 1;0 -1 0;0 0 -1;0 0 0;1 0 0;0 1 0;-1 0 0;0 0 0]  X0=0
  Out1 : Outport
  wires:
  State Space/1 -> Out1/1
  In1/1 -> State Space/1

== system airgk/uy-Control/uDynInv/Inv Rot/M ==
  ftp : Inport
  ftpdot : Inport  Port=2
  3x1mult : Subsystem  mask(3x1 Matrix Multiplication){}
      mask help:
      | Input 1   : elements of matrix X (3 by 3)
      |   Input 2   : elements of matrix Y (3 by 1)
      |   Output   : elements of matrix X*Y (3 by 1)
      mask Help:
      | <p>
      | Elements of input and output matrices are taken columnwise.
      | </p>
      mask Display: disp('Z=X*Y')
  Constant : Constant  Value=0
  Constant3 : Constant
  Demux : Demux  Outputs=2
  Demux1 : Demux  Outputs=2
  Gain : Gain  Gain=-1  SaturateOnIntegerOverflow=on  OutDataTypeStr=Inherit: Same as input  ParamDataTypeStr=Inherit: Same as input
  Gain1 : Gain  Gain=-1  SaturateOnIntegerOverflow=on  OutDataTypeStr=Inherit: Same as input  ParamDataTypeStr=Inherit: Same as input
  Mux : Mux  Inputs=9
  Product : Product  SaturateOnIntegerOverflow=on  RndMeth=Zero  InputSameDT=on  OutDataTypeStr=Inherit: Same as first input
  Product1 : Product  SaturateOnIntegerOverflow=on  RndMeth=Zero  InputSameDT=on  OutDataTypeStr=Inherit: Same as first input
  Selector : Selector  InputPortWidth=3  IndexOptions=Index vector (dialog)  Indices=[1 2]  OutputSizes=1
  Trigonometric Function1 : Trigonometry  Operator=cos
  Trigonometric Function2 : Trigonometry
  pqr : Outport
  wires:
  Constant3/1 -> Mux/1
  Constant/1 -> Mux/2, Mux/3, Mux/4
  Gain/1 -> Mux/6
  Gain1/1 -> Mux/7
  Trigonometric Function1/1 -> Demux/1
  Demux1/2 -> Gain1/1
  Product/1 -> Mux/8
  Product1/1 -> Mux/9
  Demux/2 -> Product/1, Product1/1
  Demux/1 -> Mux/5, Product1/2
  Selector/1 -> Trigonometric Function1/1, Trigonometric Function2/1
  ftpdot/1 -> 3x1mult/2(Y)
  Mux/1 -> 3x1mult/1(X)
  3x1mult/1(Z) -> pqr/1
  Trigonometric Function2/1 -> Demux1/1
  Demux1/1 -> Gain/1, Product/2
  ftp/1 -> Selector/1

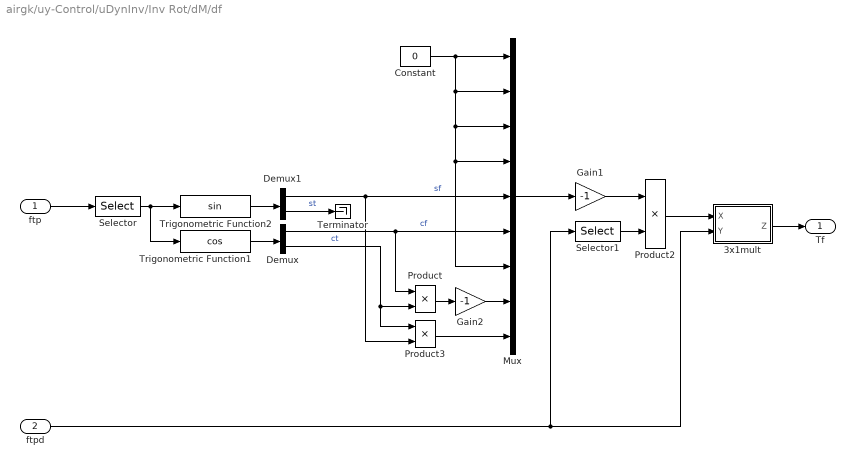
== system airgk/uy-Control/uDynInv/Inv Rot/dM/df ==
  ftp : Inport
  ftpd : Inport  Port=2
  3x1mult : Subsystem  mask(3x1 Matrix Multiplication){}
      mask help:
      | Input 1   : elements of matrix X (3 by 3)
      |   Input 2   : elements of matrix Y (3 by 1)
      |   Output   : elements of matrix X*Y (3 by 1)
      mask Help:
      | <p>
      | Elements of input and output matrices are taken columnwise.
      | </p>
      mask Display: disp('Z=X*Y')
  Constant : Constant  Value=0
  Demux : Demux  Outputs=2
  Demux1 : Demux  Outputs=2
  Gain1 : Gain  Gain=-1  SaturateOnIntegerOverflow=on  OutDataTypeStr=Inherit: Same as input  ParamDataTypeStr=Inherit: Same as input
  Gain2 : Gain  Gain=-1  SaturateOnIntegerOverflow=on  OutDataTypeStr=Inherit: Same as input  ParamDataTypeStr=Inherit: Same as input
  Mux : Mux  Inputs=9
  Product : Product  SaturateOnIntegerOverflow=on  RndMeth=Zero  InputSameDT=on  OutDataTypeStr=Inherit: Same as first input
  Product2 : Product  SaturateOnIntegerOverflow=on  RndMeth=Zero  InputSameDT=on  OutDataTypeStr=Inherit: Same as first input
  Product3 : Product  SaturateOnIntegerOverflow=on  RndMeth=Zero  InputSameDT=on  OutDataTypeStr=Inherit: Same as first input
  Selector : Selector  InputPortWidth=3  IndexOptions=Index vector (dialog)  Indices=[1 2]  OutputSizes=1
  Selector1 : Selector  InputPortWidth=3  IndexOptions=Index vector (dialog)  Indices=1  OutputSizes=1
  Terminator : Terminator
  Trigonometric Function1 : Trigonometry  Operator=cos
  Trigonometric Function2 : Trigonometry
  Tf : Outport
  wires:
  3x1mult/1(Z) -> Tf/1
  Selector1/1 -> Product2/2
  Product2/1 -> 3x1mult/1(X)
  ftpd/1 -> Selector1/1, 3x1mult/2(Y)
  Gain1/1 -> Product2/1
  Mux/1 -> Gain1/1
  Constant/1 -> Mux/3, Mux/4, Mux/7, Mux/2, Mux/1
  ftp/1 -> Selector/1
  Trigonometric Function2/1 -> Demux1/1
  Selector/1 -> Trigonometric Function2/1, Trigonometric Function1/1
  Trigonometric Function1/1 -> Demux/1
  Demux1/1 -> Mux/5, Product3/2  "sf"
  Demux/1 -> Mux/6, Product/1  "cf"
  Product/1 -> Gain2/1
  Demux/2 -> Product/2, Product3/1  "ct"
  Product3/1 -> Mux/9
  Demux1/2 -> Terminator/1  "st"
  Gain2/1 -> Mux/8

== system airgk/uy-Control/uDynInv/Inv Rot/dM/dt ==
  ftp : Inport
  ftpd : Inport  Port=2
  3x1mult : Subsystem  mask(3x1 Matrix Multiplication){}
      mask help:
      | Input 1   : elements of matrix X (3 by 3)
      |   Input 2   : elements of matrix Y (3 by 1)
      |   Output   : elements of matrix X*Y (3 by 1)
      mask Help:
      | <p>
      | Elements of input and output matrices are taken columnwise.
      | </p>
      mask Display: disp('Z=X*Y')
  Constant : Constant  Value=0
  Demux : Demux  Outputs=2
  Demux1 : Demux  Outputs=2
  Gain1 : Gain  Gain=-1  SaturateOnIntegerOverflow=on  OutDataTypeStr=Inherit: Same as input  ParamDataTypeStr=Inherit: Same as input
  Mux : Mux  Inputs=9
  Product : Product  SaturateOnIntegerOverflow=on  RndMeth=Zero  InputSameDT=on  OutDataTypeStr=Inherit: Same as first input
  Product1 : Product  SaturateOnIntegerOverflow=on  RndMeth=Zero  InputSameDT=on  OutDataTypeStr=Inherit: Same as first input
  Product2 : Product  SaturateOnIntegerOverflow=on  RndMeth=Zero  InputSameDT=on  OutDataTypeStr=Inherit: Same as first input
  Selector : Selector  InputPortWidth=3  IndexOptions=Index vector (dialog)  Indices=[1 2]  OutputSizes=1
  Selector1 : Selector  InputPortWidth=3  IndexOptions=Index vector (dialog)  Indices=2  OutputSizes=1
  Trigonometric Function1 : Trigonometry  Operator=cos
  Trigonometric Function2 : Trigonometry
  Tt : Outport
  wires:
  Trigonometric Function1/1 -> Demux/1
  Selector/1 -> Trigonometric Function2/1, Trigonometric Function1/1
  Trigonometric Function2/1 -> Demux1/1
  ftp/1 -> Selector/1
  Constant/1 -> Mux/1, Mux/2, Mux/3, Mux/4, Mux/5, Mux/6
  Demux/2 -> Mux/7  "ct"
  Product/1 -> Mux/8
  Product1/1 -> Mux/9
  Mux/1 -> Gain1/1
  Gain1/1 -> Product2/1
  Demux1/1 -> Product/1  "sf"
  Demux1/2 -> Product/2, Product1/1  "st"
  Demux/1 -> Product1/2  "cf"
  ftpd/1 -> 3x1mult/2(Y), Selector1/1
  Product2/1 -> 3x1mult/1(X)
  Selector1/1 -> Product2/2
  3x1mult/1(Z) -> Tt/1

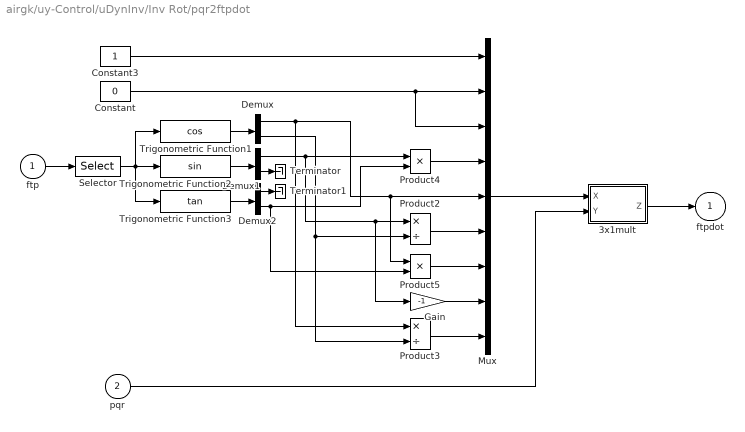
== system airgk/uy-Control/uDynInv/Inv Rot/pqr2ftpdot ==
  ftp : Inport
  pqr : Inport  Port=2
  3x1mult : Subsystem  mask(3x1 Matrix Multiplication){}
      mask help:
      | Input 1   : elements of matrix X (3 by 3)
      |   Input 2   : elements of matrix Y (3 by 1)
      |   Output   : elements of matrix X*Y (3 by 1)
      mask Help:
      | <p>
      | Elements of input and output matrices are taken columnwise.
      | </p>
      mask Display: disp('Z=X*Y')
  Constant : Constant  Value=0
  Constant3 : Constant
  Demux : Demux  Outputs=2
  Demux1 : Demux  Outputs=2
  Demux2 : Demux  Outputs=2
  Gain : Gain  Gain=-1  SaturateOnIntegerOverflow=on  OutDataTypeStr=Inherit: Same as input  ParamDataTypeStr=Inherit: Same as input
  Mux : Mux  Inputs=9
  Product2 : Product  Inputs=*/  SaturateOnIntegerOverflow=on  RndMeth=Zero  InputSameDT=on  OutDataTypeStr=Inherit: Same as first input
  Product3 : Product  Inputs=*/  SaturateOnIntegerOverflow=on  RndMeth=Zero  InputSameDT=on  OutDataTypeStr=Inherit: Same as first input
  Product4 : Product  SaturateOnIntegerOverflow=on  RndMeth=Zero  InputSameDT=on  OutDataTypeStr=Inherit: Same as first input
  Product5 : Product  SaturateOnIntegerOverflow=on  RndMeth=Zero  InputSameDT=on  OutDataTypeStr=Inherit: Same as first input
  Selector : Selector  InputPortWidth=3  IndexOptions=Index vector (dialog)  Indices=[1 2]  OutputSizes=1
  Terminator : Terminator
  Terminator1 : Terminator
  Trigonometric Function1 : Trigonometry  Operator=cos
  Trigonometric Function2 : Trigonometry
  Trigonometric Function3 : Trigonometry  Operator=tan
  ftpdot : Outport
  wires:
  3x1mult/1(Z) -> ftpdot/1
  Mux/1 -> 3x1mult/1(X)
  pqr/1 -> 3x1mult/2(Y)
  Trigonometric Function3/1 -> Demux2/1
  Constant3/1 -> Mux/1
  Constant/1 -> Mux/2, Mux/3
  Product4/1 -> Mux/4
  Trigonometric Function2/1 -> Demux1/1
  Trigonometric Function1/1 -> Demux/1
  ftp/1 -> Selector/1
  Selector/1 -> Trigonometric Function2/1, Trigonometric Function3/1, Trigonometric Function1/1
  Demux1/1 -> Product4/1, Product2/1, Gain/1
  Product5/1 -> Mux/7
  Product2/1 -> Mux/6
  Demux2/2 -> Product4/2, Product5/2
  Demux/1 -> Mux/5, Product5/1, Product3/1
  Demux/2 -> Product2/2, Product3/2
  Product3/1 -> Mux/9
  Demux1/2 -> Terminator/1
  Demux2/1 -> Terminator1/1
  Gain/1 -> Mux/8

== system airgk/uy-Control/uDynInv/ad1/0 ==

== system airgk/uy-Control/uDynInv/atm/0 ==

== system airgk/uy-Control/uDynInv/dl/0 ==

== system airgk/Subsystem/eqm/ODE/Eulerdot/0 ==

== system airgk/Subsystem/eqm/ODE/Vabdot/0 ==

== system airgk/Subsystem/eqm/ODE/pqrdot/0 ==

== system airgk/Subsystem/eqm/ODE/pqrdot/GM2  ==
  In1 : Inport
  Matrix Gain : StateSpace  A=[]  B=[]  C=[]  D=M  X0=0
  Out1 : Outport
  wires:
  In1/1 -> Matrix Gain/1
  Matrix Gain/1 -> Out1/1

== system airgk/Subsystem/eqm/ODE/xyHdot/0 ==

== system airgk/uy-Control/Vcmd Generator/xyHdot/3x1/Dot Product1 ==
  In1 : Inport
  In2 : Inport  Port=2
  S-Function : S-Function  FunctionName=sdotproduct  SFunctionDeploymentMode=off  EnableBusSupport=off
  Out1 : Outport
  wires:
  In2/1 -> S-Function/2
  In1/1 -> S-Function/1
  S-Function/1 -> Out1/1

== system airgk/uy-Control/Vcmd Generator/xyHdot/3x1/Dot Product2 ==
  In1 : Inport
  In2 : Inport  Port=2
  S-Function : S-Function  FunctionName=sdotproduct  SFunctionDeploymentMode=off  EnableBusSupport=off
  Out1 : Outport
  wires:
  S-Function/1 -> Out1/1
  In1/1 -> S-Function/1
  In2/1 -> S-Function/2

== system airgk/uy-Control/Vcmd Generator/xyHdot/3x1/Dot Product9 ==
  In1 : Inport
  In2 : Inport  Port=2
  S-Function : S-Function  FunctionName=sdotproduct  SFunctionDeploymentMode=off  EnableBusSupport=off
  Out1 : Outport
  wires:
  S-Function/1 -> Out1/1
  In1/1 -> S-Function/1
  In2/1 -> S-Function/2

== system airgk/uy-Control/uDynInv/Inv Rot/M/3x1mult ==
  X : Inport
  Y : Inport  Port=2
  Dot Product : DotProduct  OutDataTypeStr=Inherit: Inherit via internal rule
  Dot Product1 : DotProduct  OutDataTypeStr=Inherit: Inherit via internal rule
  Dot Product2 : DotProduct  OutDataTypeStr=Inherit: Inherit via internal rule
  Mux : Mux  Inputs=3
  Selector : Selector  InputPortWidth=9  IndexOptions=Index vector (dialog)  Indices=[0 3 6]+1  OutputSizes=1
  Selector1 : Selector  InputPortWidth=9  IndexOptions=Index vector (dialog)  Indices=[0 3 6]+2  OutputSizes=1
  Selector2 : Selector  InputPortWidth=9  IndexOptions=Index vector (dialog)  Indices=[0 3 6]+3  OutputSizes=1
  Z : Outport
  wires:
  Y/1 -> Dot Product/2, Dot Product1/2, Dot Product2/2
  Selector2/1 -> Dot Product2/1
  Selector1/1 -> Dot Product1/1
  Selector/1 -> Dot Product/1
  Mux/1 -> Z/1
  Dot Product2/1 -> Mux/3
  Dot Product1/1 -> Mux/2
  Dot Product/1 -> Mux/1
  X/1 -> Selector2/1, Selector1/1, Selector/1

== system airgk/uy-Control/uDynInv/Inv Rot/dM/df/3x1mult ==
  X : Inport
  Y : Inport  Port=2
  Dot Product : DotProduct  OutDataTypeStr=Inherit: Inherit via internal rule
  Dot Product1 : DotProduct  OutDataTypeStr=Inherit: Inherit via internal rule
  Dot Product2 : DotProduct  OutDataTypeStr=Inherit: Inherit via internal rule
  Mux : Mux  Inputs=3
  Selector : Selector  InputPortWidth=9  IndexOptions=Index vector (dialog)  Indices=[0 3 6]+1  OutputSizes=1
  Selector1 : Selector  InputPortWidth=9  IndexOptions=Index vector (dialog)  Indices=[0 3 6]+2  OutputSizes=1
  Selector2 : Selector  InputPortWidth=9  IndexOptions=Index vector (dialog)  Indices=[0 3 6]+3  OutputSizes=1
  Z : Outport
  wires:
  Y/1 -> Dot Product/2, Dot Product1/2, Dot Product2/2
  Selector2/1 -> Dot Product2/1
  Selector1/1 -> Dot Product1/1
  Selector/1 -> Dot Product/1
  Mux/1 -> Z/1
  Dot Product2/1 -> Mux/3
  Dot Product1/1 -> Mux/2
  Dot Product/1 -> Mux/1
  X/1 -> Selector2/1, Selector1/1, Selector/1

== system airgk/uy-Control/uDynInv/Inv Rot/dM/dt/3x1mult ==
  X : Inport
  Y : Inport  Port=2
  Dot Product : DotProduct  OutDataTypeStr=Inherit: Inherit via internal rule
  Dot Product1 : DotProduct  OutDataTypeStr=Inherit: Inherit via internal rule
  Dot Product2 : DotProduct  OutDataTypeStr=Inherit: Inherit via internal rule
  Mux : Mux  Inputs=3
  Selector : Selector  InputPortWidth=9  IndexOptions=Index vector (dialog)  Indices=[0 3 6]+1  OutputSizes=1
  Selector1 : Selector  InputPortWidth=9  IndexOptions=Index vector (dialog)  Indices=[0 3 6]+2  OutputSizes=1
  Selector2 : Selector  InputPortWidth=9  IndexOptions=Index vector (dialog)  Indices=[0 3 6]+3  OutputSizes=1
  Z : Outport
  wires:
  Y/1 -> Dot Product/2, Dot Product1/2, Dot Product2/2
  Selector2/1 -> Dot Product2/1
  Selector1/1 -> Dot Product1/1
  Selector/1 -> Dot Product/1
  Mux/1 -> Z/1
  Dot Product2/1 -> Mux/3
  Dot Product1/1 -> Mux/2
  Dot Product/1 -> Mux/1
  X/1 -> Selector2/1, Selector1/1, Selector/1

== system airgk/uy-Control/uDynInv/Inv Rot/pqr2ftpdot/3x1mult ==
  X : Inport
  Y : Inport  Port=2
  Dot Product : DotProduct  OutDataTypeStr=Inherit: Inherit via internal rule
  Dot Product1 : DotProduct  OutDataTypeStr=Inherit: Inherit via internal rule
  Dot Product2 : DotProduct  OutDataTypeStr=Inherit: Inherit via internal rule
  Mux : Mux  Inputs=3
  Selector : Selector  InputPortWidth=9  IndexOptions=Index vector (dialog)  Indices=[0 3 6]+1  OutputSizes=1
  Selector1 : Selector  InputPortWidth=9  IndexOptions=Index vector (dialog)  Indices=[0 3 6]+2  OutputSizes=1
  Selector2 : Selector  InputPortWidth=9  IndexOptions=Index vector (dialog)  Indices=[0 3 6]+3  OutputSizes=1
  Z : Outport
  wires:
  Y/1 -> Dot Product/2, Dot Product1/2, Dot Product2/2
  Selector2/1 -> Dot Product2/1
  Selector1/1 -> Dot Product1/1
  Selector/1 -> Dot Product/1
  Mux/1 -> Z/1
  Dot Product2/1 -> Mux/3
  Dot Product1/1 -> Mux/2
  Dot Product/1 -> Mux/1
  X/1 -> Selector2/1, Selector1/1, Selector/1
